simulink model "Cv_04_1"  (R2022b)
settings: Solver=VariableStepAuto  StartTime=0.0  StopTime=100.0  RelTol=1e-3
libraries: simulink x1
settings Model: Creator=honza  LastModifiedBy=honza

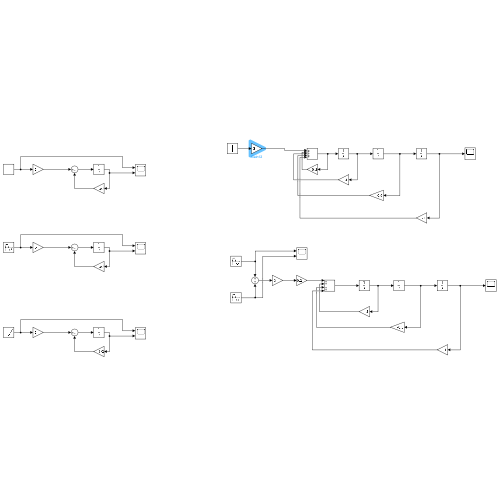
[thumbnail: Simulink's stored preview of the top-level diagram]
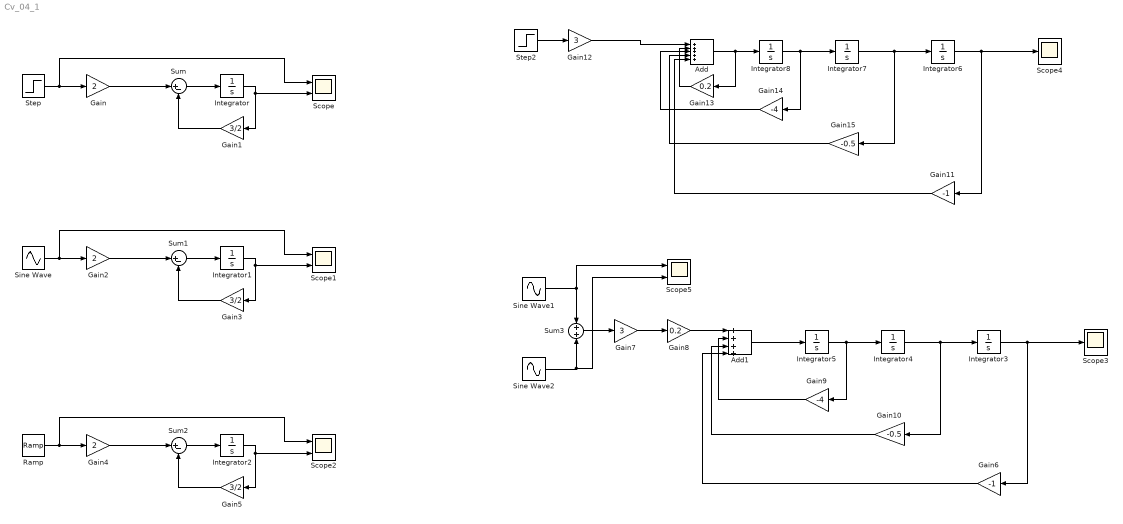
== system Cv_04_1 ==
  Add : Sum  Inputs=+++++
  Add1 : Sum  Inputs=++++
  Gain : Gain  Gain=2
  Gain1 : Gain  Gain=3/2
  Gain10 : Gain  Gain=-0.5
  Gain11 : Gain  Gain=-1
  Gain12 : Gain  Gain=3
  Gain13 : Gain  Gain=0.2
  Gain14 : Gain  Gain=-4
  Gain15 : Gain  Gain=-0.5
  Gain2 : Gain  Gain=2
  Gain3 : Gain  Gain=3/2
  Gain4 : Gain  Gain=2
  Gain5 : Gain  Gain=3/2
  Gain6 : Gain  Gain=-1
  Gain7 : Gain  Gain=3
  Gain8 : Gain  Gain=0.2
  Gain9 : Gain  Gain=-4
  Integrator{,1..8} (9 alike) : Integrator
  Ramp : simulink/Sources/Ramp  slope=1  start=0  InitialOutput=0
  Scope{,1..2,5} (4 alike) : Scope  NumInputPorts=2
  Scope3 : Scope
  Scope4 : Scope
  Sine Wave : Sin  SampleTime=0
  Sine Wave1 : Sin  SampleTime=0
  Sine Wave2 : Sin  Phase=pi/2  SampleTime=0
  Step : Step  Time=0  SampleTime=0
  Step2 : Step  SampleTime=0
  Sum : Sum  Inputs=|+-
  Sum1 : Sum  Inputs=|+-
  Sum2 : Sum  Inputs=|+-
  Sum3 : Sum  Inputs=+|+
  wires:
  Sum/1 -> Integrator/1
  Step/1 -> Scope/1, Gain/1
  Gain/1 -> Sum/1
  Gain1/1 -> Sum/2
  Integrator/1 -> Scope/2, Gain1/1
  Integrator1/1 -> Scope1/2, Gain3/1
  Gain2/1 -> Sum1/1
  Sum1/1 -> Integrator1/1
  Sine Wave/1 -> Scope1/1, Gain2/1
  Gain3/1 -> Sum1/2
  Integrator2/1 -> Scope2/2, Gain5/1
  Gain4/1 -> Sum2/1
  Sum2/1 -> Integrator2/1
  Ramp/1 -> Scope2/1, Gain4/1
  Gain5/1 -> Sum2/2
  Integrator6/1 -> Gain11/1, Scope4/1
  Integrator7/1 -> Integrator6/1, Gain15/1
  Integrator8/1 -> Integrator7/1, Gain14/1
  Step2/1 -> Gain12/1
  Gain14/1 -> Add/3
  Gain15/1 -> Add/4
  Gain11/1 -> Add/5
  Add/1 -> Gain13/1, Integrator8/1
  Add1/1 -> Integrator5/1
  Gain8/1 -> Add1/1
  Gain7/1 -> Gain8/1
  Gain6/1 -> Add1/4
  Gain10/1 -> Add1/3
  Gain9/1 -> Add1/2
  Sum3/1 -> Gain7/1
  Integrator5/1 -> Gain9/1, Integrator4/1
  Integrator4/1 -> Gain10/1, Integrator3/1
  Integrator3/1 -> Scope3/1, Gain6/1
  Sine Wave2/1 -> Scope5/2, Sum3/2
  Sine Wave1/1 -> Sum3/1, Scope5/1
  Gain13/1 -> Add/2
  Gain12/1 -> Add/1
